simulink model "simulation_scheme_pos"  (R2021b)
settings: Solver=FixedStepAuto  StartTime=0.0  StopTime=simulation.stop_time  FixedStep=simulation.step_size  RelTol=1e-5
PreLoadFcn:
  | % initialize variables
  | initializeUnicycleModel;
undefined symbols (not defined in the file): camera, controller, derivator, obstacle, park, tracking, unicycle
settings Model: Creator=beniamino  LastModifiedBy=gioel
settings SolverCC: AlgebraicLoopSolver=TrustRegion
settings DataIOCC: InitialState=cartesianInitialStates  SaveFormat=Structure

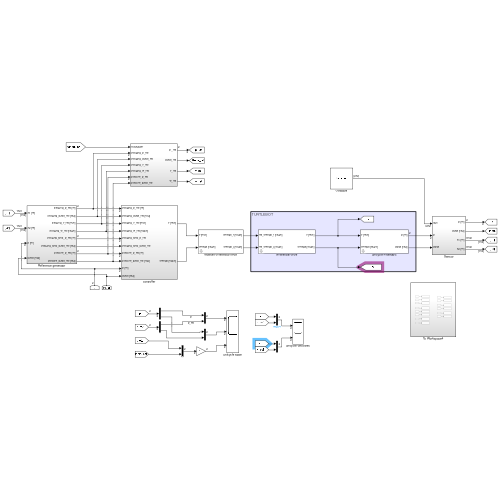
[thumbnail: Simulink's stored preview of the top-level diagram]
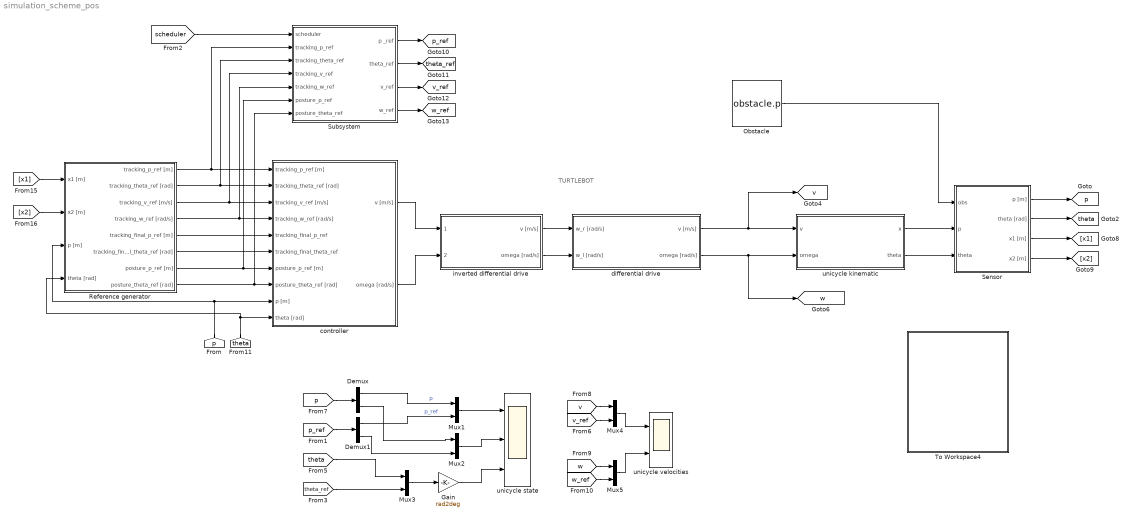
== system simulation_scheme_pos ==
  note: TURTLEBOT
  Demux : Demux  Outputs=2
  Demux1 : Demux  Outputs=2
  Gain : Gain  Gain=rad2deg
  Mux{1..5} (5 alike) : Mux  Inputs=2
  Obstacle : Constant  Value=obstacle.p
  Reference generator : Subsystem
  Sensor : Subsystem
  Subsystem : Subsystem
  To Workspace4 : Subsystem
  controller : Subsystem
  differential drive : Subsystem  mask(Differential drive for a unicycle){r=unicycle.diffDrive.r, d=unicycle.diffDrive.d, wheelDyEn=on, Tc=unicycle.diffDrive.Td, wheelsSpeedUpperLimit=unicycle.diffDrive.omegaWheelMax, wheelsSpeedLowerLimit=unicycle.diffDrive.omegaWheelMin}
      mask prompts: r "wheel radius"; d "interaxis lenght"; wheelDyEn "l.p.f. enable"; Tc "time constant [s]"; wheelsSpeedUpperLimit "max wheel speed  [rad/s]"; wheelsSpeedLowerLimit "min wheel speed [rad/s]"
      mask help:
      | Model of a differential drive.
      | It takes as input the derired wheel velocities and converts them to the corresponding driving velocity and stearing velocity.
      | Wheels dynamics can be taken into accont, along with output saturation.
      mask Help:
      | author: Beniamino Pozzan
      | email: beniamino.pozzan@phd.unipd.it
      mask Callback wheelDyEn:
      | % get the enable parameter
      | wheelDyEnStatus = get_param(gcb,'wheelDyEn');
      | enableStatus = get_param(gcb,'MaskEnables');
      | % if it is true, make Tc enabled
      | if strcmp(wheelDyEnStatus,'on')
      |     enableStatus{4}='on';
      | else
      |     enableStatus{4}='off';
      | end
      | set_param(gcb,'MaskEnables',enableStatus)
      mask TypeOptions wheelsSpeedUpperLimit: w_l saturator/UpperLimit | w_r saturator/UpperLimit
      mask TypeOptions wheelsSpeedLowerLimit: w_l saturator/LowerLimit | w_r saturator/LowerLimit
      mask DialogControl wheelDy Prompt: wheel dynamics
  inverted differential drive : Subsystem  mask(Inverted Differential drive for a unicycle){r=unicycle.diffDrive.r, d=unicycle.diffDrive.d}
      mask prompts: r "wheel radius"; d "interaxis lenght"
      mask help:
      | Inverted differential drive for a unicycle.
      | Provided the desired driving and stearing velocities, it computes the corresponding wheel velocities.
  unicycle kinematic : Subsystem  mask(Unicycle Kinematic Model){x0=unicycle.ic.x, y0=unicycle.ic.y, theta0=unicycle.ic.theta}
      mask prompts: x0 "x_0"; y0 "y_0"; theta0 "theta_0"
      mask help: kinematic model of a unicyle.
  unicycle state : Scope  NumInputPorts=3
  unicycle velocities : Scope  NumInputPorts=2
  tag scope: p=global, p_ref=global, theta=global, theta_ref=global, v=global, v_ref=global, w=global, w_ref=global
  wires:
  inverted differential drive/1(v [m/s]) -> differential drive/1(w_r [rad/s])
  inverted differential drive/2(omega [rad/s]) -> differential drive/2(w_l [rad/s])
  differential drive/1(v [m/s]) -> [v], unicycle kinematic/1(v)
  differential drive/2(omega [rad/s]) -> [w], unicycle kinematic/2(omega)
  unicycle kinematic/1(x) -> Sensor/2(p)
  unicycle kinematic/2(theta) -> Sensor/3(theta)
  [p] -> Demux/1
  [p_ref] -> Demux1/1
  Mux1/1 -> unicycle state/1
  Mux2/1 -> unicycle state/2
  Demux/1 -> Mux1/1  "p"
  Demux1/1 -> Mux1/2  "p_ref"
  Demux/2 -> Mux2/1
  Demux1/2 -> Mux2/2
  [theta] -> Mux3/1
  [theta_ref] -> Mux3/2
  Mux4/1 -> unicycle velocities/1
  Mux5/1 -> unicycle velocities/2
  [v] -> Mux4/1
  [v_ref] -> Mux4/2
  [w] -> Mux5/1
  [w_ref] -> Mux5/2
  [theta] -> Reference generator/4(theta [rad]), controller/10(theta [rad])
  controller/1(v [m/s]) -> inverted differential drive/1(1)
  controller/2(omega [rad/s]) -> inverted differential drive/2(2)
  Reference generator/1(tracking_p_ref [m]) -> Subsystem/2(tracking_p_ref), controller/1(tracking_p_ref [m])
  Reference generator/4(tracking_w_ref [rad/s]) -> Subsystem/5(tracking_w_ref), controller/4(tracking_w_ref [rad/s])
  Reference generator/5(tracking_final_p_ref [m]) -> controller/5(tracking_final_p_ref)
  Reference generator/6(tracking_final_theta_ref [rad]) -> controller/6(tracking_final_theta_ref)
  Reference generator/8(posture_theta_ref [rad]) -> Subsystem/7(posture_theta_ref), controller/8(posture_theta_ref [rad])
  Reference generator/3(tracking_v_ref [m/s]) -> Subsystem/4(tracking_v_ref), controller/3(tracking_v_ref [m/s])
  Mux3/1 -> Gain/1
  Gain/1 -> unicycle state/3
  Sensor/1(p [m]) -> [p]
  Sensor/2(theta [rad]) -> [theta]
  Sensor/3(x1 [m]) -> [x1]
  Sensor/4(x2 [m]) -> [x2]
  Obstacle/1 -> Sensor/1(obs)
  [x1] -> Reference generator/1(x1 [m])
  [x2] -> Reference generator/2(x2 [m])
  [p] -> Reference generator/3(p [m]), controller/9(p [m])
  Subsystem/4(w_ref) -> [w_ref]
  [scheduler] -> Subsystem/1(scheduler)
  Subsystem/1(p _ref) -> [p_ref]
  Reference generator/2(tracking_theta_ref [rad]) -> Subsystem/3(tracking_theta_ref), controller/2(tracking_theta_ref [rad])
  Subsystem/2(theta_ref) -> [theta_ref]
  Subsystem/3(v_ref) -> [v_ref]
  Reference generator/7(posture_p_ref [m]) -> Subsystem/6(posture_p_ref), controller/7(posture_p_ref [m])

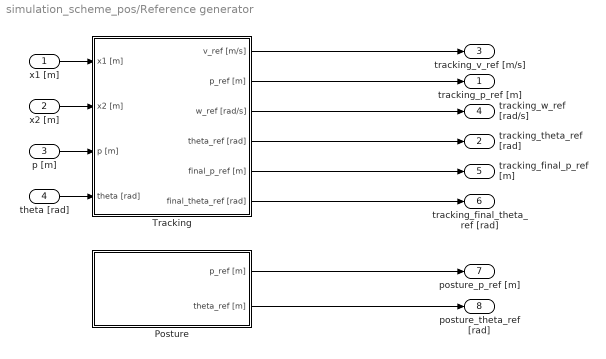
== system simulation_scheme_pos/Reference generator ==
  x1 [m] : Inport
  x2 [m] : Inport  Port=2
  p [m] : Inport  Port=3
  theta [rad] : Inport  Port=4
  Posture : Subsystem
  Tracking : Subsystem
  tracking_p_ref [m] : Outport
  tracking_theta_ref [rad] : Outport  Port=2
  tracking_v_ref [m/s] : Outport  Port=3
  tracking_w_ref [rad/s] : Outport  Port=4
  tracking_final_p_ref [m] : Outport  Port=5
  tracking_final_theta_ref [rad] : Outport  Port=6
  posture_p_ref [m] : Outport  Port=7
  posture_theta_ref [rad] : Outport  Port=8
  wires:
  Tracking/3(w_ref [rad/s]) -> tracking_w_ref [rad/s]/1
  Tracking/1(v_ref [m/s]) -> tracking_v_ref [m/s]/1
  Posture/1(p_ref [m]) -> posture_p_ref [m]/1
  Tracking/5(final_p_ref [m]) -> tracking_final_p_ref [m]/1
  Tracking/4(theta_ref [rad]) -> tracking_theta_ref [rad]/1
  Tracking/6(final_theta_ref [rad]) -> tracking_final_theta_ref [rad]/1
  Tracking/2(p_ref [m]) -> tracking_p_ref [m]/1
  Posture/2(theta_ref [m]) -> posture_theta_ref [rad]/1
  x2 [m]/1 -> Tracking/2(x2 [m])
  x1 [m]/1 -> Tracking/1(x1 [m])
  p [m]/1 -> Tracking/3(p [m])
  theta [rad]/1 -> Tracking/4(theta [rad])

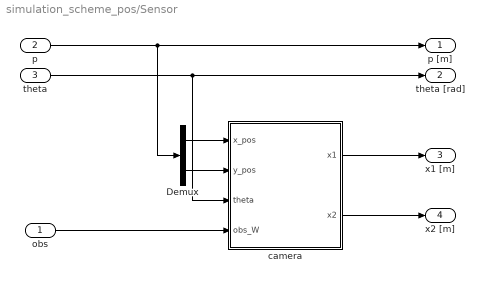
== system simulation_scheme_pos/Sensor ==
  obs : Inport
  p : Inport  Port=2
  theta : Inport  Port=3
  Demux : Demux  Outputs=2
  camera : MATLAB Function  TreatAsAtomicUnit=on
  p [m] : Outport
  theta [rad] : Outport  Port=2
  x1 [m] : Outport  Port=3
  x2 [m] : Outport  Port=4
  wires:
  theta/1 -> camera/3(theta), theta [rad]/1
  obs/1 -> camera/4(obs_W)
  p/1 -> Demux/1, p [m]/1
  Demux/1 -> camera/1(x_pos)
  Demux/2 -> camera/2(y_pos)
  camera/1(x1) -> x1 [m]/1
  camera/2(x2) -> x2 [m]/1

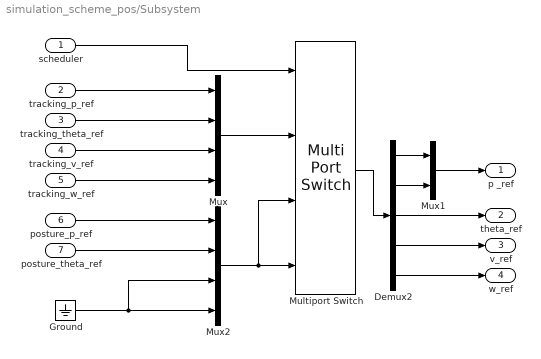
== system simulation_scheme_pos/Subsystem ==
  scheduler : Inport
  tracking_p_ref : Inport  Port=2
  tracking_theta_ref : Inport  Port=3
  tracking_v_ref : Inport  Port=4
  tracking_w_ref : Inport  Port=5
  posture_p_ref : Inport  Port=6
  posture_theta_ref : Inport  Port=7
  Demux2 : Demux  Outputs=5
  Ground : Ground
  Multiport Switch : MultiPortSwitch
  Mux : Mux
  Mux1 : Mux  Inputs=2
  Mux2 : Mux
  p _ref : Outport
  theta_ref : Outport  Port=2
  v_ref : Outport  Port=3
  w_ref : Outport  Port=4
  wires:
  tracking_theta_ref/1 -> Mux/2
  scheduler/1 -> Multiport Switch/1
  tracking_p_ref/1 -> Mux/1
  Multiport Switch/1 -> Demux2/1
  Mux/1 -> Multiport Switch/2
  Ground/1 -> Mux2/3, Mux2/4
  tracking_v_ref/1 -> Mux/3
  tracking_w_ref/1 -> Mux/4
  Mux2/1 -> Multiport Switch/3, Multiport Switch/4
  posture_p_ref/1 -> Mux2/1
  posture_theta_ref/1 -> Mux2/2
  Demux2/1 -> Mux1/1
  Demux2/2 -> Mux1/2
  Mux1/1 -> p _ref/1
  Demux2/3 -> theta_ref/1
  Demux2/4 -> v_ref/1
  Demux2/5 -> w_ref/1

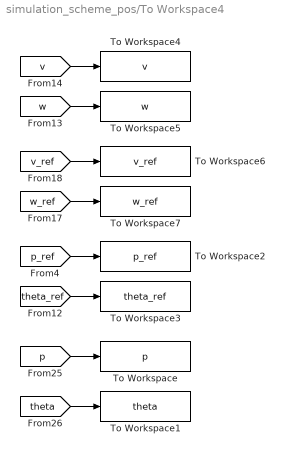
== system simulation_scheme_pos/To Workspace4 ==
  To Workspace : ToWorkspace  VariableName=p  SaveFormat=Timeseries  SampleTime=-1
  To Workspace1 : ToWorkspace  VariableName=theta  SaveFormat=Timeseries  SampleTime=-1
  To Workspace2 : ToWorkspace  VariableName=p_ref  SaveFormat=Timeseries  SampleTime=-1
  To Workspace3 : ToWorkspace  VariableName=theta_ref  SaveFormat=Timeseries  SampleTime=-1
  To Workspace4 : ToWorkspace  VariableName=v  SaveFormat=Timeseries  SampleTime=-1
  To Workspace5 : ToWorkspace  VariableName=w  SaveFormat=Timeseries  SampleTime=-1
  To Workspace6 : ToWorkspace  VariableName=v_ref  SaveFormat=Timeseries  SampleTime=-1
  To Workspace7 : ToWorkspace  VariableName=w_ref  SaveFormat=Timeseries  SampleTime=-1
  wires:
  [v_ref] -> To Workspace6/1
  [w_ref] -> To Workspace7/1
  [theta] -> To Workspace1/1
  [v] -> To Workspace4/1
  [w] -> To Workspace5/1
  [p_ref] -> To Workspace2/1
  [theta_ref] -> To Workspace3/1
  [p] -> To Workspace/1

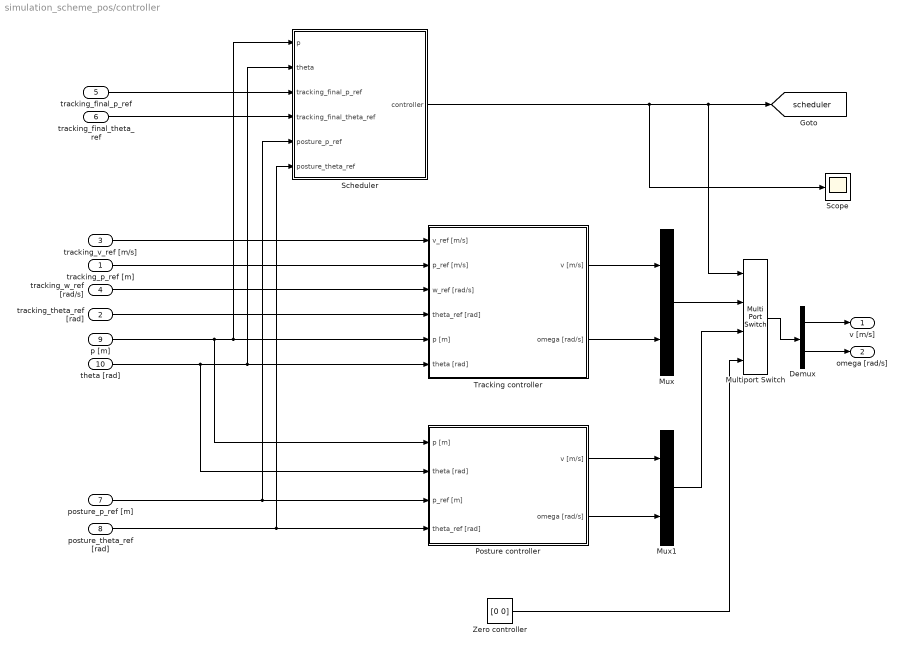
== system simulation_scheme_pos/controller ==
  tracking_p_ref [m] : Inport
  tracking_theta_ref [rad] : Inport  Port=2
  tracking_v_ref [m/s] : Inport  Port=3
  tracking_w_ref [rad/s] : Inport  Port=4
  tracking_final_p_ref : Inport  Port=5
  tracking_final_theta_ref : Inport  Port=6
  posture_p_ref [m] : Inport  Port=7
  posture_theta_ref [rad] : Inport  Port=8
  p [m] : Inport  Port=9
  theta [rad] : Inport  Port=10
  Demux : Demux  Outputs=2
  Multiport Switch : MultiPortSwitch
  Mux : Mux  Inputs=2
  Mux1 : Mux  Inputs=2
  Posture controller : Subsystem
  Scheduler : MATLAB Function  TreatAsAtomicUnit=on
  Scope : Scope
  Tracking controller : Subsystem
  Zero controller : Constant  Value=[0 0]
  v [m/s] : Outport
  omega [rad/s] : Outport  Port=2
  tag scope: scheduler=global
  wires:
  Multiport Switch/1 -> Demux/1
  Tracking controller/1(v [m/s]) -> Mux/1
  Tracking controller/2(omega [rad/s]) -> Mux/2
  Demux/2 -> omega [rad/s]/1
  Demux/1 -> v [m/s]/1
  Mux/1 -> Multiport Switch/2
  tracking_p_ref [m]/1 -> Tracking controller/2(p_ref [m/s])
  tracking_theta_ref [rad]/1 -> Tracking controller/4(theta_ref [rad])
  p [m]/1 -> Tracking controller/5(p [m]), Scheduler/1(p), Posture controller/1(p [m])
  Zero controller/1 -> Multiport Switch/4
  Mux1/1 -> Multiport Switch/3
  Posture controller/2(omega [rad/s]) -> Mux1/2
  Posture controller/1(v [m/s]) -> Mux1/1
  Scheduler/1(controller) -> Scope/1, Multiport Switch/1, [scheduler]
  theta [rad]/1 -> Tracking controller/6(theta [rad]), Scheduler/2(theta), Posture controller/2(theta [rad])
  posture_p_ref [m]/1 -> Posture controller/3(p_ref [m]), Scheduler/5(posture_p_ref)
  posture_theta_ref [rad]/1 -> Scheduler/6(posture_theta_ref), Posture controller/4(theta_ref [rad])
  tracking_final_p_ref/1 -> Scheduler/3(tracking_final_p_ref)
  tracking_final_theta_ref/1 -> Scheduler/4(tracking_final_theta_ref)
  tracking_v_ref [m/s]/1 -> Tracking controller/1(v_ref [m/s])
  tracking_w_ref [rad/s]/1 -> Tracking controller/3(w_ref [rad/s])

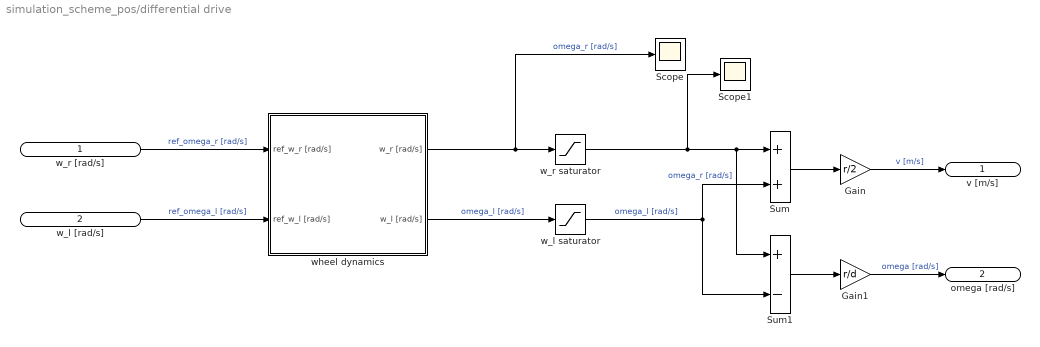
== system simulation_scheme_pos/differential drive ==
  w_r [rad/s] : Inport  Unit=rad/s
  w_l [rad/s] : Inport  Port=2  Unit=rad/s
  Gain : Gain  Gain=r/2
  Gain1 : Gain  Gain=r/d
  Scope : Scope
  Scope1 : Scope
  Sum : Sum
  Sum1 : Sum  Inputs=+-
  w_l saturator : Saturate  UpperLimit=wheelsSpeedUpperLimit  LowerLimit=wheelsSpeedLowerLimit
  w_r saturator : Saturate  UpperLimit=wheelsSpeedUpperLimit  LowerLimit=wheelsSpeedLowerLimit
  wheel dynamics : Subsystem  Variant=on
  v [m/s] : Outport  Unit=m/s
  omega [rad/s] : Outport  Port=2  Unit=rad/s
  wires:
  w_l saturator/1 -> Sum1/2, Sum/2  "omega_l [rad/s]"
  w_r saturator/1 -> Scope1/1, Sum1/1, Sum/1  "omega_r [rad/s]"
  Gain1/1 -> omega [rad/s]/1  "omega [rad/s]"
  Sum1/1 -> Gain1/1
  Gain/1 -> v [m/s]/1  "v [m/s]"
  Sum/1 -> Gain/1
  w_r [rad/s]/1 -> wheel dynamics/1(ref_w_r [rad/s])  "ref_omega_r [rad/s]"
  w_l [rad/s]/1 -> wheel dynamics/2(ref_w_l [rad/s])  "ref_omega_l [rad/s]"
  wheel dynamics/1(w_r [rad/s]) -> Scope/1, w_r saturator/1  "omega_r [rad/s]"
  wheel dynamics/2(w_l [rad/s]) -> w_l saturator/1  "omega_l [rad/s]"

== system simulation_scheme_pos/inverted differential drive ==
  1 : Inport  Unit=m/s
  2 : Inport  Port=2  Unit=rad/s
  Gain : Gain  Gain=1/r
  Gain1 : Gain  Gain=1/r
  Gain2 : Gain  Gain=d/2
  Sum : Sum
  Sum1 : Sum  Inputs=+-
  v [m/s] : Outport  Unit=rad/s
  omega [rad/s] : Outport  Port=2  Unit=rad/s
  wires:
  Gain2/1 -> Sum1/2, Sum/2
  Sum/1 -> Gain/1
  Gain/1 -> v [m/s]/1  "omega_r [rad/s]"
  Sum1/1 -> Gain1/1
  Gain1/1 -> omega [rad/s]/1  "omega_l [rad/s]"
  1/1 -> Sum1/1, Sum/1  "v [m/s]"
  2/1 -> Gain2/1  "omega [rad/s]"

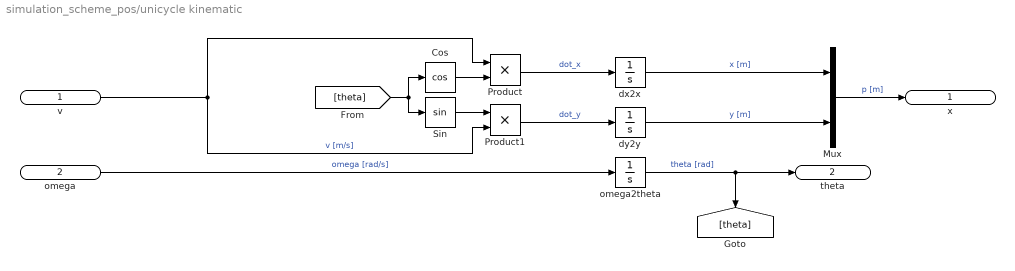
== system simulation_scheme_pos/unicycle kinematic ==
  v : Inport  PortDimensions=1
  omega : Inport  Port=2  PortDimensions=1
  Cos : Trigonometry  Operator=cos
  Mux : Mux  Inputs=2
  Product : Product
  Product1 : Product
  Sin : Trigonometry
  dx2x : Integrator  InitialCondition=x0  ContinuousStateAttributes='pos_x'
  dy2y : Integrator  InitialCondition=y0  ContinuousStateAttributes='pos_y'
  omega2theta : Integrator  InitialCondition=theta0  ContinuousStateAttributes='theta'
  x : Outport  PortDimensions=2
  theta : Outport  Port=2  PortDimensions=1
  wires:
  Product1/1 -> dy2y/1  "dot_y"
  [theta] -> Sin/1, Cos/1
  v/1 -> Product/1, Product1/2  "v [m/s]"
  omega2theta/1 -> [theta], theta/1  "theta [rad]"
  omega/1 -> omega2theta/1  "omega [rad/s]"
  dy2y/1 -> Mux/2  "y [m]"
  Cos/1 -> Product/2
  dx2x/1 -> Mux/1  "x [m]"
  Sin/1 -> Product1/1
  Product/1 -> dx2x/1  "dot_x"
  Mux/1 -> x/1  "p [m]"

== system simulation_scheme_pos/Reference generator/Posture ==
  Constant : Constant  Value=park.y  SampleTime=unicycle.diffDrive.Td
  Constant1 : Constant  Value=park.x  SampleTime=unicycle.diffDrive.Td
  Constant2 : Constant  Value=park.theta  SampleTime=unicycle.diffDrive.Td
  Mux : Mux  Inputs=2
  p_ref [m] : Outport
  theta_ref [m] : Outport  Port=2
  wires:
  Mux/1 -> p_ref [m]/1
  Constant1/1 -> Mux/1
  Constant/1 -> Mux/2
  Constant2/1 -> theta_ref [m]/1

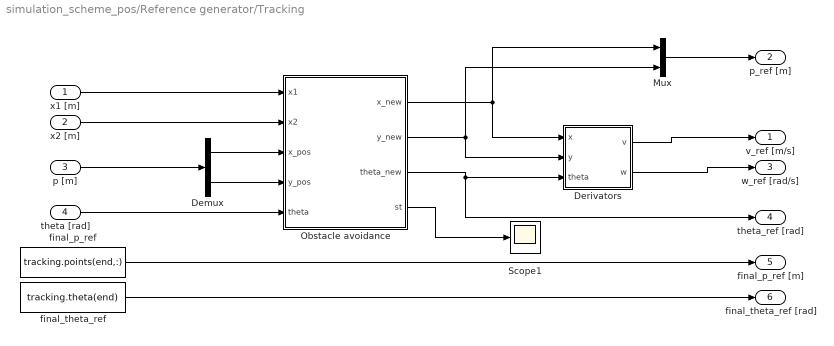
== system simulation_scheme_pos/Reference generator/Tracking ==
  x1 [m] : Inport
  x2 [m] : Inport  Port=2
  p [m] : Inport  Port=3
  theta [rad] : Inport  Port=4
  Demux : Demux  Outputs=2
  Derivators : Subsystem
  Mux : Mux  Inputs=2
  Obstacle avoidance : MATLAB Function  TreatAsAtomicUnit=on
  Scope1 : Scope
  final_p_ref : Constant  Value=tracking.points(end,:)
  final_theta_ref : Constant  Value=tracking.theta(end)
  v_ref [m/s] : Outport
  p_ref [m] : Outport  Port=2
  w_ref [rad/s] : Outport  Port=3
  theta_ref [rad] : Outport  Port=4
  final_p_ref [m] : Outport  Port=5
  final_theta_ref [rad] : Outport  Port=6
  wires:
  final_p_ref/1 -> final_p_ref [m]/1
  final_theta_ref/1 -> final_theta_ref [rad]/1
  x1 [m]/1 -> Obstacle avoidance/1(x1)
  x2 [m]/1 -> Obstacle avoidance/2(x2)
  theta [rad]/1 -> Obstacle avoidance/5(theta)
  Demux/1 -> Obstacle avoidance/3(x_pos)
  Demux/2 -> Obstacle avoidance/4(y_pos)
  p [m]/1 -> Demux/1
  Mux/1 -> p_ref [m]/1
  Obstacle avoidance/1(x_new) -> Mux/1, Derivators/1(x)
  Obstacle avoidance/2(y_new) -> Mux/2, Derivators/2(y)
  Obstacle avoidance/3(theta_new) -> theta_ref [rad]/1, Derivators/3(theta)
  Derivators/1(v) -> v_ref [m/s]/1
  Derivators/2(w) -> w_ref [rad/s]/1
  Obstacle avoidance/4(st) -> Scope1/1

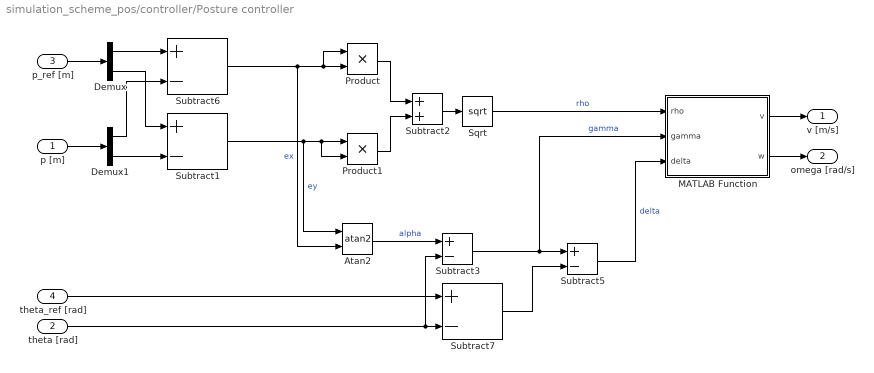
== system simulation_scheme_pos/controller/Posture controller ==
  p [m] : Inport
  theta [rad] : Inport  Port=2
  p_ref [m] : Inport  Port=3
  theta_ref [rad] : Inport  Port=4
  Atan2 : Trigonometry  Operator=atan2
  Demux : Demux  Outputs=2
  Demux1 : Demux  Outputs=2
  MATLAB Function : MATLAB Function  TreatAsAtomicUnit=on
  Product : Product
  Product1 : Product
  Sqrt : Sqrt  SaturateOnIntegerOverflow=on
  Subtract{1,3,5..7} (5 alike) : Sum  Inputs=+-
  Subtract2 : Sum
  v [m/s] : Outport
  omega [rad/s] : Outport  Port=2
  wires:
  p_ref [m]/1 -> Demux/1
  p [m]/1 -> Demux1/1
  Subtract6/1 -> Atan2/2, Product/1, Product/2  "ex"
  Subtract1/1 -> Product1/1, Product1/2, Atan2/1  "ey"
  Product1/1 -> Subtract2/2
  Product/1 -> Subtract2/1
  Subtract2/1 -> Sqrt/1
  Sqrt/1 -> MATLAB Function/1(rho)  "rho"
  Subtract3/1 -> Subtract5/1, MATLAB Function/2(gamma)  "gamma"
  theta [rad]/1 -> Subtract7/2, Subtract3/2
  MATLAB Function/1(v) -> v [m/s]/1
  MATLAB Function/2(w) -> omega [rad/s]/1
  Subtract5/1 -> MATLAB Function/3(delta)  "delta"
  Atan2/1 -> Subtract3/1  "alpha"
  Demux/1 -> Subtract6/1
  Demux1/1 -> Subtract6/2
  Demux/2 -> Subtract1/1
  Demux1/2 -> Subtract1/2
  theta_ref [rad]/1 -> Subtract7/1
  Subtract7/1 -> Subtract5/2

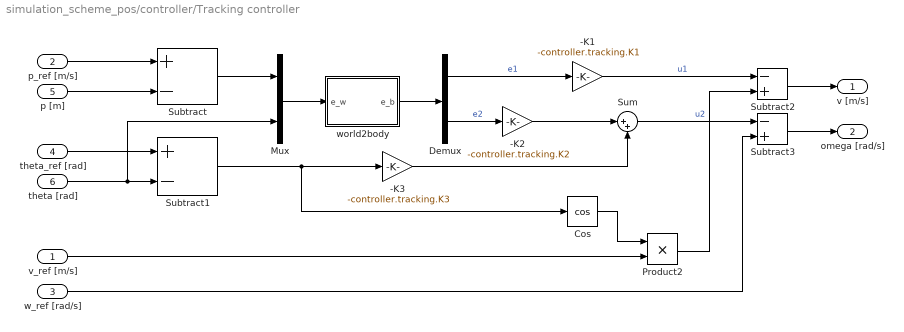
== system simulation_scheme_pos/controller/Tracking controller ==
  v_ref [m/s] : Inport
  p_ref [m/s] : Inport  Port=2
  w_ref [rad/s] : Inport  Port=3
  theta_ref [rad] : Inport  Port=4
  p [m] : Inport  Port=5
  theta [rad] : Inport  Port=6
  -K1 : Gain  Gain=-controller.tracking.K1
  -K2 : Gain  Gain=-controller.tracking.K2
  -K3 : Gain  Gain=-controller.tracking.K3
  Cos : Trigonometry  Operator=cos
  Demux : Demux  Outputs=2
  Mux : Mux  Inputs=2
  Product2 : Product
  Subtract : Sum  Inputs=+-
  Subtract1 : Sum  Inputs=+-
  Subtract2 : Sum  Inputs=-+
  Subtract3 : Sum  Inputs=-+
  Sum : Sum  Inputs=|++
  world2body : MATLAB Function  TreatAsAtomicUnit=on
  v [m/s] : Outport
  omega [rad/s] : Outport  Port=2
  wires:
  Subtract2/1 -> v [m/s]/1
  -K1/1 -> Subtract2/1  "u1"
  theta [rad]/1 -> Mux/2, Subtract1/2
  p [m]/1 -> Subtract/2
  Subtract/1 -> Mux/1
  Demux/2 -> -K2/1  "e2"
  -K2/1 -> Sum/1
  Subtract3/1 -> omega [rad/s]/1
  Mux/1 -> world2body/1(e_w)
  Cos/1 -> Product2/1
  theta_ref [rad]/1 -> Subtract1/1
  -K3/1 -> Sum/2
  Sum/1 -> Subtract3/1  "u2"
  Demux/1 -> -K1/1  "e1"
  Product2/1 -> Subtract2/2
  world2body/1(e_b) -> Demux/1
  Subtract1/1 -> Cos/1, -K3/1
  p_ref [m/s]/1 -> Subtract/1
  v_ref [m/s]/1 -> Product2/2
  w_ref [rad/s]/1 -> Subtract3/2

== system simulation_scheme_pos/differential drive/wheel dynamics ==
  ref_w_r [rad/s] : Inport
  ref_w_l [rad/s] : Inport  Port=2
  lpf : Subsystem  VariantControl=wheelDyEn==true
  none : Subsystem  VariantControl=wheelDyEn==false
  w_r [rad/s] : Outport
  w_l [rad/s] : Outport  Port=2

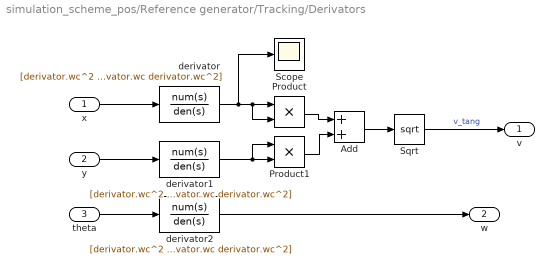
== system simulation_scheme_pos/Reference generator/Tracking/Derivators ==
  x : Inport
  y : Inport  Port=2
  theta : Inport  Port=3
  Add : Sum
  Product : Product
  Product1 : Product
  Scope : Scope
  Sqrt : Sqrt  SaturateOnIntegerOverflow=on
  derivator : TransferFcn  Numerator=[derivator.wc^2 0]  Denominator=[1 2*derivator.delta*derivator.wc derivator.wc^2]
  derivator1 : TransferFcn  Numerator=[derivator.wc^2 0]  Denominator=[1 2*derivator.delta*derivator.wc derivator.wc^2]
  derivator2 : TransferFcn  Numerator=[derivator.wc^2 0]  Denominator=[1 2*derivator.delta*derivator.wc derivator.wc^2]
  v : Outport
  w : Outport  Port=2
  wires:
  x/1 -> derivator/1
  Sqrt/1 -> v/1  "v_tang"
  derivator/1 -> Scope/1, Product/2, Product/1
  derivator1/1 -> Product1/2, Product1/1
  Add/1 -> Sqrt/1
  Product/1 -> Add/1
  Product1/1 -> Add/2
  y/1 -> derivator1/1
  theta/1 -> derivator2/1
  derivator2/1 -> w/1

== system simulation_scheme_pos/differential drive/wheel dynamics/lpf ==
  ref_w_r [rad/s] : Inport
  ref_w_l [rad/s] : Inport  Port=2
  w_r_lpf : TransferFcn  Denominator=[Tc 1]  ContinuousStateAttributes='w_r_lpf'
  w_r_lpf1 : TransferFcn  Denominator=[Tc 1]  ContinuousStateAttributes='w_r_lpf'
  w_r [rad/s] : Outport
  w_l [rad/s] : Outport  Port=2
  wires:
  ref_w_r [rad/s]/1 -> w_r_lpf/1
  w_r_lpf1/1 -> w_l [rad/s]/1  "w_r [rad/s]"
  w_r_lpf/1 -> w_r [rad/s]/1  "w_l [rad/s]"
  ref_w_l [rad/s]/1 -> w_r_lpf1/1  "w_r [rad/s]"

== system simulation_scheme_pos/differential drive/wheel dynamics/none ==
  ref_w_r [rad/s] : Inport
  ref_w_l [rad/s] : Inport  Port=2
  w_r [rad/s] : Outport
  w_l [rad/s] : Outport  Port=2
  wires:
  ref_w_r [rad/s]/1 -> w_r [rad/s]/1  "w_l [rad/s]"
  ref_w_l [rad/s]/1 -> w_l [rad/s]/1  "w_r [rad/s]"

== matlab function simulation_scheme_pos/controller/Tracking controller/world2body ==
  data: e_w input; e_b output
function e_b = fcn(e_w)

%
% This function expresses the position and orientation error wrt RF_B
%
% Inputs:
% e_w    : e_w = [e_x; e_y; e_theta] wrt RF_W
%
% Outputs:
% e_b    : e_b = [e_x; e_y; e_theta] wrt RF_B

e_b = [cos(e_w(3)) sin(e_w(3)); -sin(e_w(3)) cos(e_w(3))] * [e_w(1); e_w(2)];

== matlab function simulation_scheme_pos/controller/Scheduler ==
  settings: updateMethod=DISCRETE  sampleTime=unicycle.diffDrive.Td
  data: p input; theta input; controller output; tracking_final_p_ref input; tracking_final_theta_ref input; posture_p_ref input; posture_theta_ref input; scheduler parameter
function controller  =  fcn(p, theta, tracking_final_p_ref, tracking_final_theta_ref, ...
      posture_p_ref, posture_theta_ref, scheduler)

%
% This function returns the index of the active controller
% (tracking controller : index = 1, posture controller : index = 2, no controller : index = 3)
% When the agent is close enough to the end of the tracking reference signal --> switch controller
%
% Inputs:
% p                        : current position of the agent
% theta                    : current orientation of the agent
% tracking_final_p_ref     : final tracking reference position
% tracking_final_theta_ref : final tracking reference orientation
% posture_p_ref            : parking place position
% posture_theta_ref        : parking place orientation
%
% Outputs:
% controller               : index of the active controller

% state: index of the active controller
% 1 - tracking controller
% 2 - posture controller
% 3 - zero controller
persistent state;

% inizialition
if isempty(state)
   state = 1;
end

switch state
    case 1

        % Check if the agent reaches the end of the track
        if (norm(p-tracking_final_p_ref) <= scheduler.threshold_p) && ...
           (abs(theta-tracking_final_theta_ref) <= scheduler.threshold_theta)
            state = 2;
        end
    
    case 2

        % Check if the agent reaches the desired position
        if (norm(p-posture_p_ref) <= scheduler.threshold_p) && ...
           (abs(theta-posture_theta_ref) <= scheduler.threshold_theta) 
            state = 3;
        end
    
    case 3

        % Do nothing
end

% Return the index of the active controller
controller = state;

end

== matlab function simulation_scheme_pos/controller/Posture controller/MATLAB Function ==
  data: rho input; gamma input; delta input; v output; w output; controller parameter
function [v,w] = fcn(rho, gamma, delta, controller)

%
% This function computes the feedback control law acting on v, w
%
% Inputs:
% rho   : length of the error vector
% delta : atan2(y_pos, x_pos) + pi
% gamma : delta - theta
%
% Outputs:
% v     : linear velocity
% w     : angular velocity

v = controller.posture.Kv * rho * cos(gamma);
w = controller.posture.Kw * gamma + controller.posture.Kv * ... 
    sin(gamma) * cos(gamma) / gamma * (gamma + ...
    controller.posture.Kdelta * delta);

== matlab function simulation_scheme_pos/Sensor/camera ==
  settings: updateMethod=DISCRETE  sampleTime=0.01
  data: x_pos input; x1 output; x2 output; y_pos input; theta input; obs_W input; camera parameter; unicycle parameter
function [x1, x2] = fcn(x_pos, y_pos, theta, obs_W, camera, unicycle)

%
% This function returns the image plane coordinate x1, x2 of camera C1 and C2, 
% respectively, given one or more obstacles expressed wrt RF_W.
%
% Inputs:
% x_pos: x coordinate of the agent wrt RF_W
% y_pos: y coordinate of the agent wrt RF_W
% theta: orientation of the agent
% obs_W: position of one or more obstacles wrt RF_W
%
% Outputs:
% x1: Camera1 image plane coordinate --> its size depends on the number of obstacles
% x2: Camera2 image plane coordinate --> its size depends on the number of obstacles

% Rotation matrix definition
R_WB = [cos(theta) -sin(theta); sin(theta) cos(theta)]; % Body to World
R_CW = transpose(R_WB*unicycle.R_BC); % World to Camera

% Translation matrix definition
T_WB = [x_pos;y_pos];

% Express obstacle in C1,C2 RFs
obs_C1 = R_CW*obs_W - transpose(unicycle.R_BC)*unicycle.T_BC1 - R_CW*T_WB;
obs_C2 = R_CW*obs_W - transpose(unicycle.R_BC)*unicycle.T_BC2 - R_CW*T_WB;

[~,num_obs] = size(obs_W); % Number of obstacles
x1 = zeros(1,num_obs);
x2 = zeros(1,num_obs);

% Iterate through number of obstacles
for i = 1:num_obs

    if obs_C1(2,i) > camera.focal_length && norm(obs_C1(:,i)) < camera.depth && ...
       atan2(obs_C1(2,i), obs_C1(1,i)) >= - camera.fov && ...
       atan2(obs_C1(2,i), obs_C1(1,i)) <= camera.fov

       % Obstacle in C1 image plane
       x1(i) = camera.focal_length*(obs_C1(1,i)/obs_C1(2,i));
    else
       x1(i) = nan;
    end
    if obs_C2(2,i) > camera.focal_length && norm(obs_C2(:,i)) < camera.depth && ...
       atan2(obs_C2(2,i), obs_C2(1,i)) >= - camera.fov && ...
       atan2(obs_C2(2,i), obs_C2(1,i)) <= camera.fov

       % Obstacle in C2 image plane
       x2(i) = camera.focal_length*(obs_C2(1,i)/obs_C2(2,i));
    else
        x2(i) = nan;
    end

end

== matlab function simulation_scheme_pos/Reference generator/Tracking/Obstacle avoidance ==
  settings: updateMethod=DISCRETE  sampleTime=0.01
  data: x1 input; x_new output; y_new output; theta_new output; x2 input; x_pos input; y_pos input; theta input; tracking parameter; unicycle parameter; st output; camera parameter
function [x_new, y_new, theta_new, st] = fcn(x1, x2, x_pos, y_pos, theta, tracking, unicycle, camera)

%
% The following obstacle avoidance method works when the obstacle is 
% placed both at a curvilenear and straight stretch.
% When the obstacle is / obstacles are detected and the closest one to the
% agent is at a dangerous distance then the overcoming manouver is computed
% as an interpolation between the initial point, the final point and
% a point chosen at a given distance 'tracking.obstacle_distance' from the
% obstacle.
% The agent overcomes the obstacle by steering always first to the left
%
% Inputs:
% x1          : camera1 image plane coordinate / coordinates
% x2          : camera2 image plane coordinate / coordinates
% x_pos       : x-coordinate of the agent wrt RF_W
% y_pos       : y-coordinate of the agent wrt RF_W
% theta       : orientation of the agent
%
% Outputs:
% x_new       : new x-coordinate reference tracking signal
% y_new       : new y-coordinate reference tracking signal
% theta_new   : new orientation reference tracking signal
% st          : state

% Length of the overcoming path
overcoming_path_length = 700;

% state = 1 if tracking reference
% state = -1 if overcoming obstacle
persistent state

% Overcoming path
persistent x_ref
persistent y_ref
persistent theta_ref

persistent k1 % Current time instant - tracking
persistent k2 % Current time instant - overcoming

persistent final_k1; % Time at which the tracking procedure restarts

if isempty(k1)
    state = 1;
    x_ref = zeros(1,overcoming_path_length);
    y_ref = zeros(1,overcoming_path_length);
    theta_ref = zeros(1,overcoming_path_length);
    k1 = 1;
    k2 = overcoming_path_length;
    final_k1 = 1;
end

if state == 1
    
    % Number of obstacles
    [~,num_obs] = size(x1);
    
    % Express obstacles wrt RF_C1 and consider the closest one to the agent
    min_dist = 100;
    p_W = [nan; nan]; % Obstacle wrt RF_W
    py_C1 = nan; % Obstacle wrt RF_C1
    px_C1 = nan;
    for i = 1:num_obs
        if(not(isnan(x1(i))) && not(isnan(x2(i))))

            % Triangulation
            curr_py_C1 = unicycle.b * camera.focal_length / (x1(i) - x2(i));
            curr_px_C1 = x1(i) * unicycle.b / (x1(i) - x2(i));
            curr_p_C1 = [curr_px_C1;curr_py_C1]; % Obstacle wrt RF_C1
            curr_p_B = unicycle.R_BC * curr_p_C1 + unicycle.T_BC1; % Obstacle wrt RF_B

            % Obstacle wrt RF_W
            R_WB = [cos(theta) -sin(theta); sin(theta) cos(theta)]; % Rotation matrix from body to world
            T_WB = [x_pos;y_pos]; % Translation matrix
            curr_p_W = R_WB * curr_p_B + T_WB;
            
            % Find closest obstacle
            dist = norm([x_pos; y_pos] - curr_p_W);
            if dist < min_dist
                min_dist = dist;
                p_W = curr_p_W;
                py_C1 = curr_py_C1;
                px_C1 = curr_px_C1;
            end
        end
    end
    
    if(not(isnan(p_W(1))) && not(isnan(p_W(2))))

        % Check if the closest obstacle is too near
        % If the obstacle is too near, modify the path
        if py_C1 > camera.focal_length && py_C1 <= unicycle.dangerous_distance && px_C1 < 0.6 && px_C1 > -0.4

            % Start overcoming procedure which takes place until k2 <= overcoming_path_length
            state = -1;
            k2 = 1;
           
            % Find the position in the path nearest to the obstacle
            [~,obs_index] = min(vecnorm([tracking.x; tracking.y] - p_W));
           
            % Time at which the overcoming procedure ends
            final_k1 = 2 * obs_index - k1 + round((obs_index - k1)/3);

            %final_k1 = 2 * obs_index - k1;

            % Overcoming path planning
            p_i = [tracking.x(k1); tracking.y(k1)]; % Starting point
            p_f = [tracking.x(final_k1); tracking.y(final_k1)]; % Final point


            % Orientation of the reference path at obs_index
            theta_o = tracking.theta(obs_index);

            % Translation vector
            t_theta = theta_o + pi/2;
            t = [tracking.distance_obstacle * cos(t_theta); tracking.distance_obstacle * sin(t_theta)];

            % Point of the new path near the obstacle 
            p_o = p_W + t;

            % Derivatives at i and f
            xder_i = tracking.x(k1)-tracking.x(k1-1);
            yder_i = tracking.y(k1)-tracking.y(k1-1);
            xder_f = tracking.x(final_k1)-tracking.x(final_k1-1);
            yder_f = tracking.y(final_k1)-tracking.y(final_k1-1);

            % Fath from i to f
            time_instants = [1,floor(overcoming_path_length/2),overcoming_path_length];
            time = 1:1:overcoming_path_length;
            new_path = [spline(time_instants, [xder_i p_i(1) p_o(1) p_f(1) xder_f], time); ...
            spline(time_instants, [yder_i p_i(2) p_o(2) p_f(2) yder_f], time)];

            x_ref = new_path(1,:);
            y_ref = new_path(2,:);
            theta_ref = atan2(diff(y_ref), diff(x_ref));
            theta_ref = cat(2, theta_ref, [theta_ref(end)]); % Padding

            for i=2:length(theta_ref)
                if theta_ref(i) - theta_ref(i-1) > 350*pi/180
                    theta_ref(i) = theta_ref(i) - 2*pi;
                elseif theta_ref(i) - theta_ref(i-1) < -350*pi/180
                    theta_ref(i) = theta_ref(i) + 2*pi;
                end
            end
           
        end
    end
end

% Tracking original reference
if state == 1

    if k1 <= length(tracking.x)
        theta_new = tracking.theta(k1);
        x_new = tracking.x(k1);
        y_new = tracking.y(k1);
        k1 = k1 + 1;
    else

        theta_new = tracking.theta(end);
        x_new = tracking.x(end);
        y_new = tracking.y(end);
    end

% Tracking new reference
else

    theta_new = theta_ref(k2);
    x_new = x_ref(k2);
    y_new = y_ref(k2);
    k2 = k2 + 1;

    if k2 == overcoming_path_length
        state = 1;
        k1 = final_k1 +1;
    end
end

st = state;
